simulink model "CANreceive"  (R2016b)
settings: Solver=FixedStepDiscrete  StartTime=0.0  StopTime=10.0  FixedStep=1e-3  RelTol=1e-3
libraries: mbed_lib x7
settings Model: Creator=EW  LastModifiedBy=oh
settings DataIOCC: LimitDataPoints=on  SaveFormat=Array
settings OptimizationCC: LifeSpan=1
settings DebuggingCC: SFUnexpectedBacktrackingDiag=warning  SFNoUnconditionalDefaultTransitionDiag=warning  SFExecutionAtInitializationDiag=none
settings HardwareCC: ProdBitPerPointer=32  ProdBitPerSizeT=32  ProdBitPerPtrDiffT=32  ProdLargestAtomicInteger=Long  ProdLargestAtomicFloat=Double  ProdIntDivRoundTo=Undefined  ProdWordSize=32  ProdHWDeviceType=ARM Compatible->ARM Cortex
settings ModelReferenceCC: PropagateSignalLabelsOutOfModel=off
settings RTWCC: SystemTargetFile=mbed.tlc  TemplateMakefile=mbed.tmf  Description=Mbed Target (Embedded Target)  TargetLang=C++
settings CodeAppCC: IgnoreCustomStorageClasses=off
settings STFCustomTargetCC: TargetLibSuffix=.a  GenerateSampleERTMain=on  CombineOutputUpdateFcns=on  ERTCustomFileBanners=on  SupportContinuousTime=off  SupportNonInlinedSFcns=off  RemoveResetFunc=on  MATLABClassNameForMDSCustomization=Simulink.SoftwareTarget.ERTCustomization  GRTInterface=off  SystemTargetFile=mbed.tlc
settings ERTTargetCC: GenerateSampleERTMain=on  ParMdlRefBuildCompliant=off  CompOptLevelCompliant=off  ConcurrentExecutionCompliant=off  ERTFirstTimeCompliant=off  ModelStepFunctionPrototypeControlCompliant=off  CPPClassGenCompliant=off  UseToolchainInfoCompliant=off  ERTCustomFileTemplate=mbed_file_process.tlc  ConvertIfToSwitch=off  SuppressUnreachableDefaultCases=off
settings ConfigComp: CovMetricSettings=dw  CovHtmlReporting=on  CovSaveCumulativeToWorkspaceVar=on  CovSaveSingleToWorkspaceVar=on  CovExternalEMLEnable=off

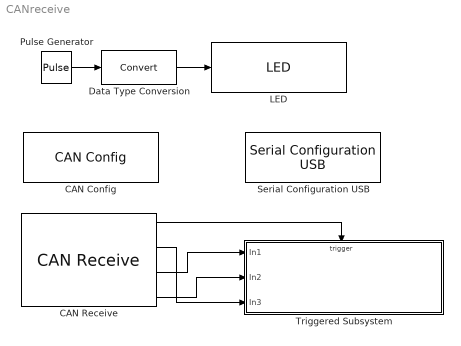
== system CANreceive ==
  CAN Config : mbed_lib/Serial/CAN/CAN Config  CAN_ID=1  CAN_frequency=1000000  CAN_Td_Port=A  CAN_Td_Pin=12  CAN_Rd_Port=A  CAN_Rd_Pin=11
  CAN Receive : mbed_lib/Serial/CAN/CAN Receive  CAN_ID=1  SampleTime=0.001
  Data Type Conversion : DataTypeConversion
  LED : mbed_lib/GPIO/LED  nLED=1  SampleTime=-1
  Pulse Generator : DiscretePulseGenerator  PulseType=Time based  Period=1  PulseWidth=50
  Serial Configuration USB : mbed_lib/Serial/UART/Serial Configuration USB  BaudRate=9600
  Triggered Subsystem : Subsystem  TreatAsAtomicUnit=on
  wires:
  CAN Receive/3 -> Triggered Subsystem/1(In1)
  CAN Receive/4 -> Triggered Subsystem/2(In2)
  CAN Receive/2 -> Triggered Subsystem/3(In3)
  CAN Receive/1 -> Triggered Subsystem/Trigger
  Pulse Generator/1 -> Data Type Conversion/1
  Data Type Conversion/1 -> LED/1

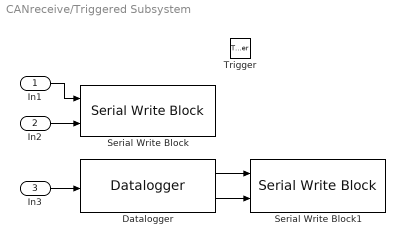
== system CANreceive/Triggered Subsystem ==
  In1 : Inport
  In2 : Inport  Port=2
  In3 : Inport  Port=3
  Trigger : TriggerPort  VariantControl=Variant
  Datalogger : mbed_lib/Utilities/Datalogger  TypeInputPorts={ 'uint16' 1 }  TypeOfInputs={'1*uint16'}  BufferSize=100  errEn=off  SampleTime=-1
  Serial Write Block : mbed_lib/Serial/UART/Serial Write Block  Priority=2  SerialPort=0  numData=on  SampleTime=-1
  Serial Write Block1 : mbed_lib/Serial/UART/Serial Write Block  Priority=1  SerialPort=0  numData=on  SampleTime=-1
  wires:
  In1/1 -> Serial Write Block/1
  In2/1 -> Serial Write Block/2
  Datalogger/2 -> Serial Write Block1/2
  In3/1 -> Datalogger/1
  Datalogger/1 -> Serial Write Block1/1
